simulink model "Super4"  (Simulink 5.0)
settings: Solver=ode45  StartTime=0.0  StopTime=10.0  RelTol=1e-3
settings Model: Creator=scaife  LastModifiedBy=scaife  ExtModeAutoUpdateStatusClock=off

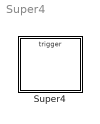
== system Super4 ==
  Super4 : Stateflow chart

== stateflow chart Super4 ==
  state A
    state A1
    (default) -> A1
  state B
    state B1
    (default) -> B1
  state C
  state D
  C -> A1 : E
  A1 -> B1 : E
  B1 -> A1 : F
  B1 -> D : E
  D -> C : E
  A -> B : G
  B -> A : G
  (default) -> C
  A1 -> C : F
  D -> B1 : F
  C -> D : F
  events: E input EITHER_EDGE_EVENT; G input EITHER_EDGE_EVENT; F input EITHER_EDGE_EVENT
